simulink model "DM"  (R2024a)
settings: Solver=VariableStepAuto  StartTime=0.0  StopTime=10.0  RelTol=1e-3
libraries: dspsigops x1, dspsrcs4 x1
settings Model: Creator=abhin  LastModifiedBy=abhin

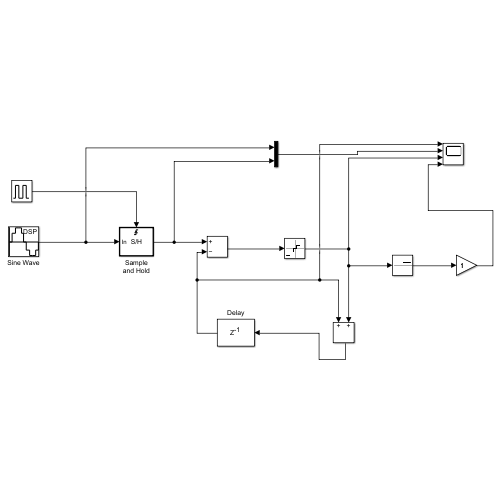
[thumbnail: Simulink's stored preview of the top-level diagram]
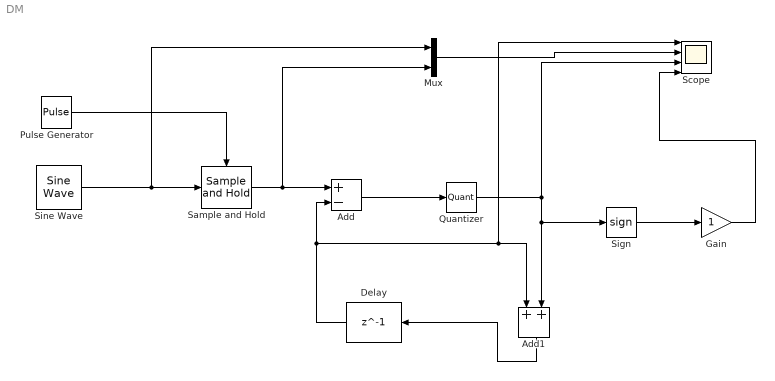
== system DM ==
  Add : Sum  Inputs=+-
  Add1 : Sum
  Delay : Delay  DelayLength=1  InitialCondition=0  UseCircularBuffer=on
  Gain : Gain
  Mux : Mux  Inputs=2
  Pulse Generator : DiscretePulseGenerator  PulseType=Time based  Period=10  PulseWidth=5
  Quantizer : Quantizer
  Sample and Hold : dspsigops/Sample and Hold  trig=Rising edge  initCond=0  latchinput=off
  Scope : Scope  NumInputPorts=4
  Sign : Signum
  Sine Wave : dspsrcs4/Sine Wave  Amplitude=1  Frequency=100  Phase=0  SampleMode=Discrete  OutComplex=Real  CompMethod=Trigonometric fcn  TableSize=Speed  SampleTime=1/1000  SamplesPerFrame=1  ResetState=Restart at time zero  OutputFrames=off  dataType=double  wordLen=16  udDataType=sfix(16)  fracBitsMode=Best precision  numFracBits=15  OutDataTypeStr=double  LastOutDataTypeStr=double
  wires:
  Sign/1 -> Gain/1
  Pulse Generator/1 -> Sample and Hold/Trigger
  Sine Wave/1 -> Mux/1, Sample and Hold/1
  Sample and Hold/1 -> Mux/2, Add/1
  Add/1 -> Quantizer/1
  Quantizer/1 -> Add1/2, Sign/1, Scope/3
  Gain/1 -> Scope/4
  Mux/1 -> Scope/2
  Add1/1 -> Delay/1
  Delay/1 -> Scope/1, Add1/1, Add/2
